simulink model "State_Feedback_Simulation"  (R2021b)
settings: Solver=VariableStepAuto  StartTime=0.0  StopTime=20  RelTol=1e-3
undefined symbols (not defined in the file): Ad, Bd, Cd, ki, Kp, L, Ts
libraries: cstblocks x1
settings Model: Creator=UTENTE  LastModifiedBy=UTENTE

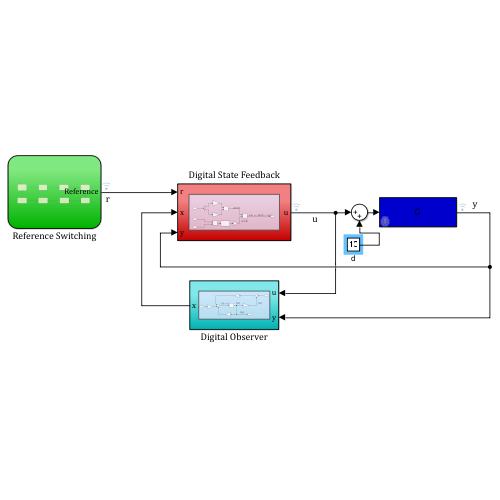
[thumbnail: Simulink's stored preview of the top-level diagram]
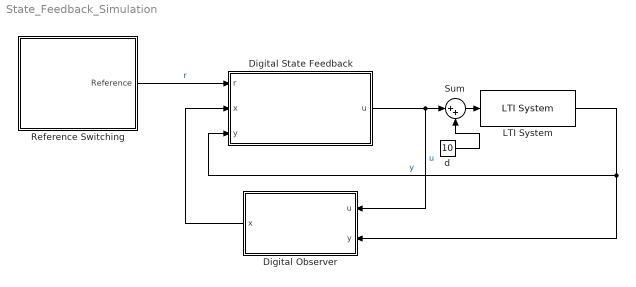
== system State_Feedback_Simulation ==
  Digital Observer : Subsystem
  Digital State Feedback : Subsystem
  LTI System : cstblocks/LTI System  sys=G  IC=[]
  Reference Switching : Stateflow chart  TreatAsAtomicUnit=on
  Sum : Sum  Inputs=|++
  d : Constant  Value=10
  wires:
  Digital State Feedback/1(u) -> Sum/1, Digital Observer/1(u)  "u"
  LTI System/1 -> Digital Observer/2(y), Digital State Feedback/3(y)  "y"
  Digital Observer/1(x) -> Digital State Feedback/2(x)
  Reference Switching/1(Reference) -> Digital State Feedback/1(r)  "r"
  Sum/1 -> LTI System/1
  d/1 -> Sum/2

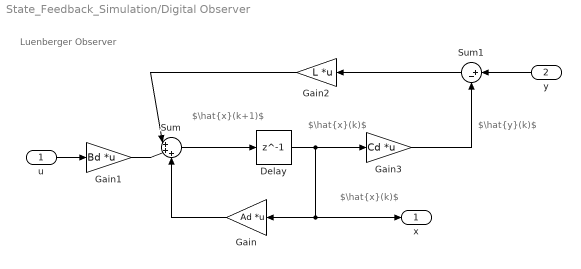
== system State_Feedback_Simulation/Digital Observer ==
  note: $\hat{x}(k+1)$
  note: Luenberger Observer
  note: $\hat{x}(k)$
  note: $\hat{y}(k)$
  note: $\hat{x}(k)$
  u : Inport
  y : Inport  Port=2
  Delay : Delay  DelayLength=1  SampleTime=Ts
  Gain : Gain  Gain=Ad  Multiplication=Matrix(K*u)
  Gain1 : Gain  Gain=Bd  Multiplication=Matrix(K*u)
  Gain2 : Gain  Gain=L  Multiplication=Matrix(K*u)
  Gain3 : Gain  Gain=Cd  Multiplication=Matrix(K*u)
  Sum : Sum  Inputs=|+++
  Sum1 : Sum  Inputs=|+-
  x : Outport
  wires:
  u/1 -> Gain1/1
  Gain3/1 -> Sum1/2
  Delay/1 -> x/1, Gain/1, Gain3/1
  Gain1/1 -> Sum/2
  Gain2/1 -> Sum/1
  Sum/1 -> Delay/1
  Gain/1 -> Sum/3
  Sum1/1 -> Gain2/1
  y/1 -> Sum1/1

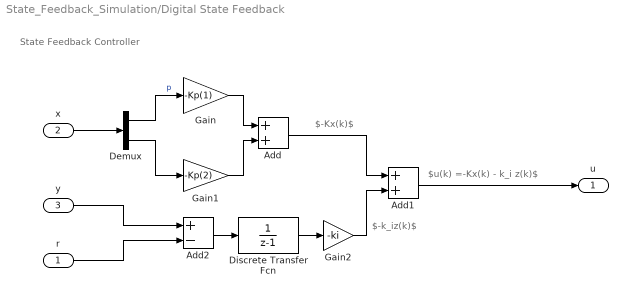
== system State_Feedback_Simulation/Digital State Feedback ==
  note: $u(k) =-Kx(k) - k_i z(k)$
  note: $-k_iz(k)$
  note: $-Kx(k)$
  note: State Feedback Controller
  r : Inport
  x : Inport  Port=2
  y : Inport  Port=3
  Add : Sum
  Add1 : Sum
  Add2 : Sum  Inputs=+-
  Demux : Demux  Outputs=2
  Discrete Transfer Fcn : DiscreteTransferFcn  Denominator=[1 -1]  SampleTime=Ts
  Gain : Gain  Gain=-Kp(1)
  Gain1 : Gain  Gain=-Kp(2)
  Gain2 : Gain  Gain=-ki
  u : Outport
  wires:
  Gain/1 -> Add/1
  y/1 -> Add2/1
  Discrete Transfer Fcn/1 -> Gain2/1
  Gain2/1 -> Add1/2
  Add2/1 -> Discrete Transfer Fcn/1
  x/1 -> Demux/1
  r/1 -> Add2/2
  Demux/2 -> Gain1/1
  Gain1/1 -> Add/2
  Add1/1 -> u/1
  Add/1 -> Add1/1
  Demux/1 -> Gain/1  "p"

== stateflow chart State_Feedback_Simulation/Reference Switching ==
  state S1
    Reference=0;
  state S2
    Reference=80;
  state S3
    Reference=125;
  state s7
    Reference=-125;
  state s6
    Reference=-80;
  state s5
    Reference=0;
  (default) -> S1
  S1 -> S2 : after(2,sec)
  S2 -> S3 : after(2,sec)
  S3 -> s5 : after(2,sec)
  s7 -> S1 : after(2,sec)
  s6 -> s7 : after(2,sec)
  s5 -> s6 : after(2,sec)
  data: Reference output
